simulink model "yek_alef_liang"  (R2024a)
settings: Solver=VariableStepAuto  StartTime=0.0  StopTime=9000  RelTol=1e-3
settings Model: Creator=MAHDI  LastModifiedBy=ASUS
settings SolverCC: AlgebraicLoopSolver=TrustRegion
settings DebuggingCC: UnconnectedInputMsg=warning  UnconnectedOutputMsg=warning  UnconnectedLineMsg=warning
settings ModelReferenceCC: EnableRefExpFcnMdlSchedulingChecks=on
settings RTWCC: GPUComputeCapability=3.5

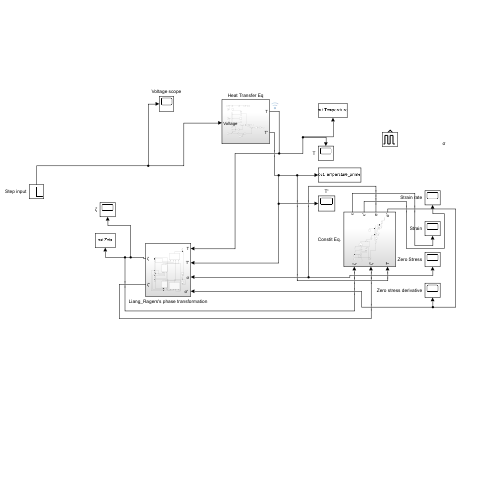
[thumbnail: Simulink's stored preview of the top-level diagram]
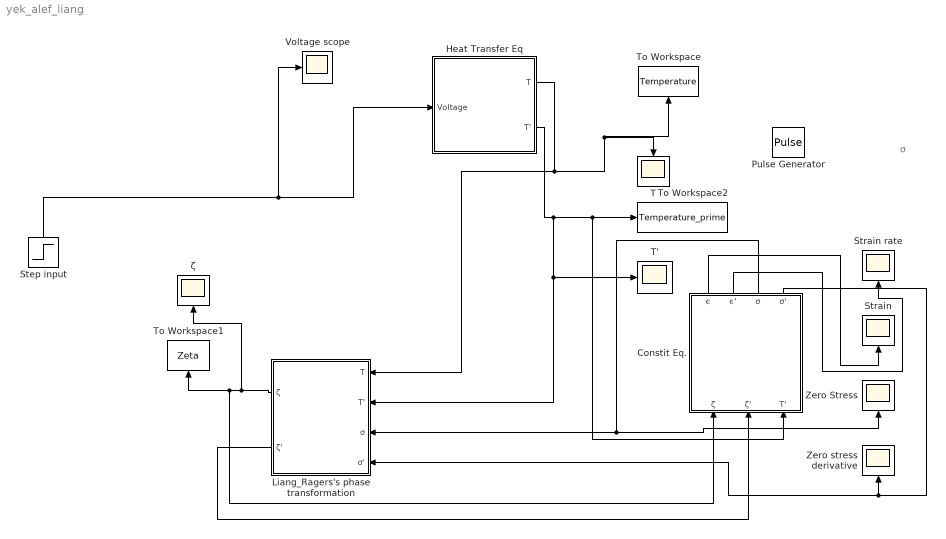
== system yek_alef_liang ==
  note: σ
  Constit Eq. : Subsystem
  Heat Transfer Eq : Subsystem
  Liang_Ragers's phase transformation : Subsystem
  Pulse Generator : DiscretePulseGenerator  PulseType=Time based  Period=100  PulseWidth=5
  Step input : Step  Time=70  Before=1  After=0  SampleTime=0
  Strain : Scope
  Strain rate : Scope
  T : Scope
  T' : Scope
  To Workspace : ToWorkspace  VariableName=Temperature  SampleTime=1
  To Workspace1 : ToWorkspace  VariableName=Zeta  SampleTime=1
  To Workspace2 : ToWorkspace  VariableName=Temperature_prime  SampleTime=1
  Voltage scope : Scope
  Zero Stress : Scope
  Zero stress derivative : Scope
  ζ : Scope
  wires:
  Heat Transfer Eq/1(T) -> To Workspace/1, T/1, Liang_Ragers's phase transformation/1(T)
  Constit Eq./1(ϵ) -> Strain/1
  Step input/1 -> Heat Transfer Eq/1(Voltage), Voltage scope/1
  Heat Transfer Eq/2(T') -> Constit Eq./3(T'), To Workspace2/1, Liang_Ragers's phase transformation/2(T'), T'/1
  Liang_Ragers's phase transformation/1(ζ) -> Constit Eq./1(ζ), To Workspace1/1, ζ/1
  Liang_Ragers's phase transformation/2(ζ') -> Constit Eq./2(ζ')
  Constit Eq./2(ϵ') -> Strain rate/1
  Constit Eq./3(σ) -> Zero Stress/1, Liang_Ragers's phase transformation/3(σ)
  Constit Eq./4(σ') -> Liang_Ragers's phase transformation/4("σ' "), Zero stress derivative/1

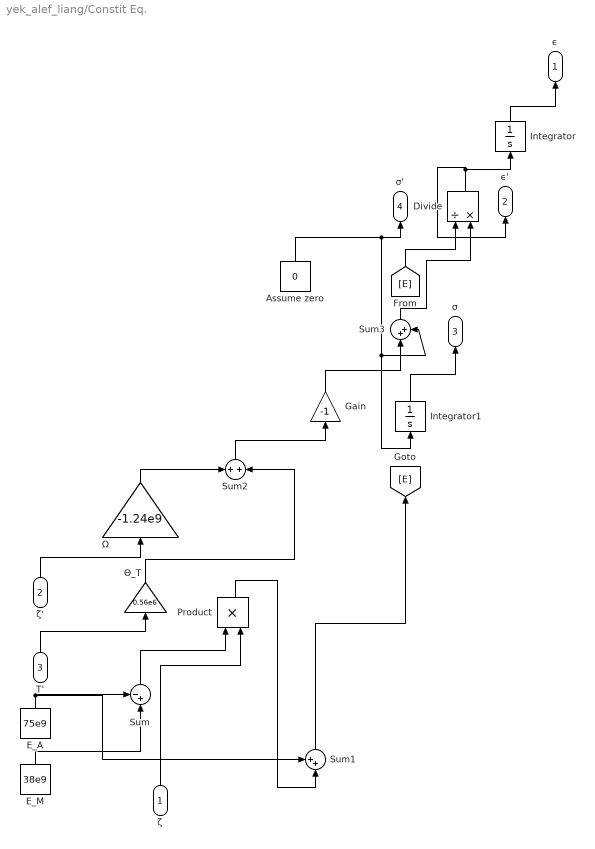
== system yek_alef_liang/Constit Eq. ==
  ζ : Inport
  ζ' : Inport  Port=2
  T' : Inport  Port=3
  Assume zero : Constant  Value=0
  Divide : Product  Inputs=/*
  E_A : Constant  Value=75e9
  E_M : Constant  Value=38e9
  Gain : Gain  Gain=-1
  Integrator : Integrator
  Integrator1 : Integrator
  Product : Product
  Sum : Sum  Inputs=-+|
  Sum1 : Sum  Inputs=++|
  Sum2 : Sum  Inputs=+|+
  Sum3 : Sum  Inputs=|++
  Θ_T : Gain  Gain=0.56e6
  Ω : Gain  Gain=-1.24e9
  ϵ : Outport
  ϵ' : Outport  Port=2
  σ : Outport  Port=3
  σ' : Outport  Port=4
  wires:
  ζ'/1 -> Ω/1
  [E] -> Divide/1
  T'/1 -> Θ_T/1
  Sum3/1 -> Divide/2
  Sum/1 -> Product/1
  E_A/1 -> Sum/1, Sum1/1
  Sum1/1 -> [E]
  Sum2/1 -> Gain/1
  E_M/1 -> Sum/2
  Divide/1 -> ϵ'/1, Integrator/1
  Θ_T/1 -> Sum2/2
  Ω/1 -> Sum2/1
  ζ/1 -> Product/2
  Product/1 -> Sum1/2
  Integrator1/1 -> σ/1
  Assume zero/1 -> Integrator1/1, Sum3/2, σ'/1
  Gain/1 -> Sum3/1
  Integrator/1 -> ϵ/1

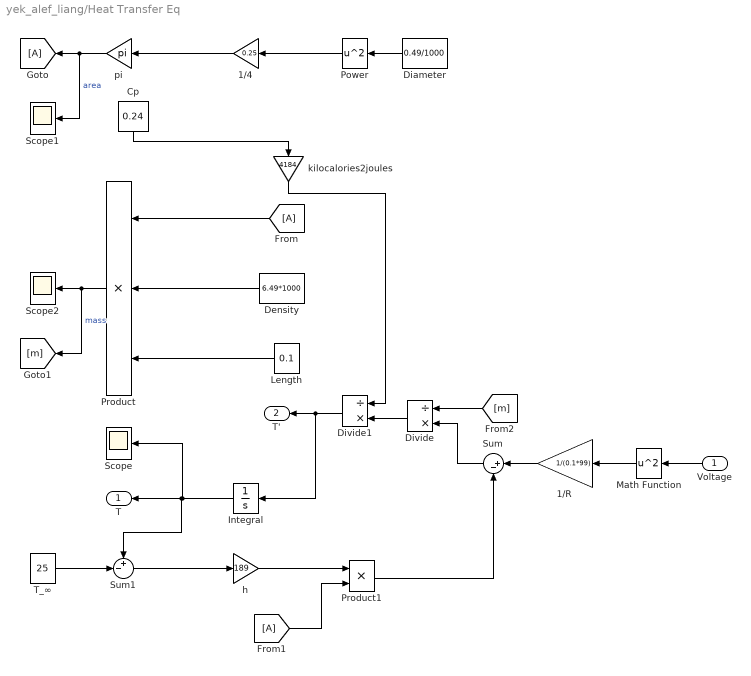
== system yek_alef_liang/Heat Transfer Eq ==
  Voltage : Inport
  1/4 : Gain  Gain=0.25
  1/R : Gain  Gain=1/(0.1*99)
  Cp : Constant  Value=0.24
  Density : Constant  Value=6.49*1000
  Diameter : Constant  Value=0.49/1000
  Divide : Product  Inputs=/*
  Divide1 : Product  Inputs=/*
  From : From
  From1 : From
  Goto : Goto
  Integral : Integrator  InitialCondition=25
  Length : Constant  Value=0.1
  Math Function : Math  Operator=square
  Power : Math  Operator=square
  Product : Product  Inputs=3
  Product1 : Product
  Scope : Scope
  Scope1 : Scope
  Scope2 : Scope
  Sum : Sum  Inputs=|+-
  Sum1 : Sum  Inputs=+-|
  T_∞ : Constant  Value=25
  h : Gain  Gain=189
  "kilocalories2joules " : Gain  Gain=4184
  pi : Gain  Gain=pi
  T : Outport
  T' : Outport  Port=2
  wires:
  Sum/1 -> Divide/2
  Sum1/1 -> h/1
  T_∞/1 -> Sum1/2
  "kilocalories2joules "/1 -> Divide1/1
  Power/1 -> 1/4/1
  Product/1 -> Scope2/1, [m]  "mass"
  pi/1 -> Goto/1, Scope1/1  "area"
  Divide/1 -> Divide1/2
  Diameter/1 -> Power/1
  Divide1/1 -> T'/1, Integral/1
  Cp/1 -> "kilocalories2joules "/1
  1/4/1 -> pi/1
  [m] -> Divide/1
  From/1 -> Product/1
  1/R/1 -> Sum/1
  Density/1 -> Product/2
  Length/1 -> Product/3
  Integral/1 -> Sum1/1, T/1, Scope/1
  Math Function/1 -> 1/R/1
  Product1/1 -> Sum/2
  h/1 -> Product1/1
  From1/1 -> Product1/2
  Voltage/1 -> Math Function/1

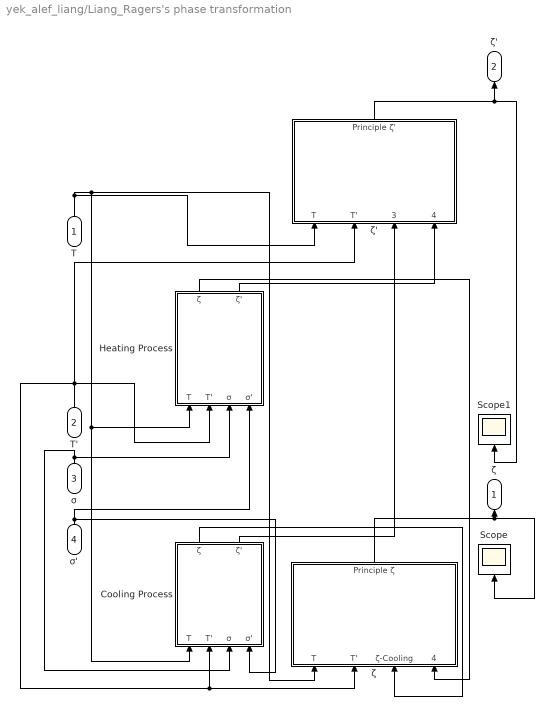
== system yek_alef_liang/Liang_Ragers's phase transformation ==
  T : Inport
  T' : Inport  Port=2
  σ : Inport  Port=3
  "σ' " : Inport  Port=4
  " ζ" : Subsystem
  " ζ'" : Subsystem
  Cooling Process : Subsystem
  Heating Process : Subsystem
  Scope : Scope
  Scope1 : Scope
  ζ : Outport
  ζ' : Outport  Port=2
  wires:
  T'/1 -> " ζ"/2(T'), Cooling Process/2(T'), " ζ'"/2(T'), Heating Process/2(T')
  Heating Process/1(ζ) -> " ζ"/4(ζ- Heating)
  "σ' "/1 -> Cooling Process/4("σ' "), Heating Process/4("σ' ")
  " ζ"/1(Principle ζ) -> ζ/1, Scope/1
  σ/1 -> Cooling Process/3(σ), Heating Process/3(σ)
  T/1 -> Cooling Process/1(T), Heating Process/1(T), " ζ"/1(T), " ζ'"/1(T)
  Heating Process/2(ζ') -> " ζ'"/4(ζ'-Heating)
  Cooling Process/1(ζ) -> " ζ"/3(ζ-Cooling)
  Cooling Process/2(ζ') -> " ζ'"/3(ζ'-Cooling)
  " ζ'"/1(Principle ζ') -> ζ'/1, Scope1/1

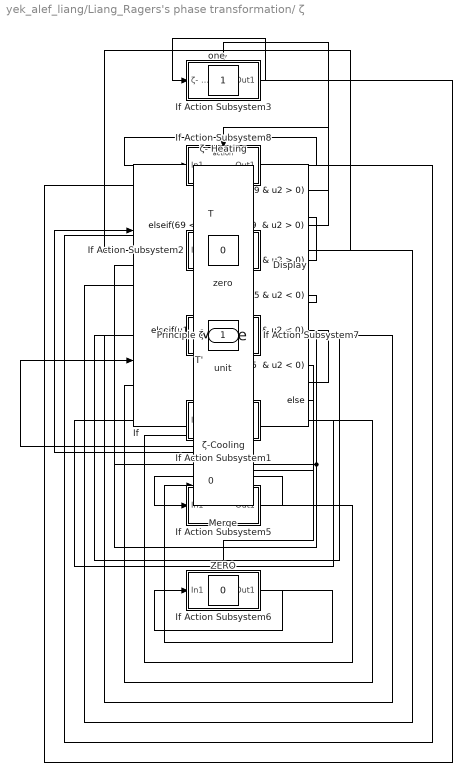
== system yek_alef_liang/Liang_Ragers's phase transformation/ ζ ==
  T : Inport
  T' : Inport  Port=2
  ζ-Cooling : Inport  Port=3
  ζ- Heating : Inport  Port=4
  0 : Constant  Value=0
  Display : Display
  If : If  NumInputs=2  IfExpression=u1 < 69 & u2 > 0  ElseIfExpressions="69 < u1 & u1 < 79  & u2 > 0 , u1 > 79 & u2 > 0 , u1 < 45 & u2 < 0 , u1 > 45 & u1 < 55 & u2 < 0 , u1 > 55  & u2 < 0"
  If Action Subsystem1 : Subsystem  TreatAsAtomicUnit=on
  If Action Subsystem2 : Subsystem  TreatAsAtomicUnit=on
  If Action Subsystem3 : Subsystem  TreatAsAtomicUnit=on
  If Action Subsystem5 : Subsystem  TreatAsAtomicUnit=on
  If Action Subsystem6 : Subsystem  TreatAsAtomicUnit=on
  If Action Subsystem7 : Subsystem  TreatAsAtomicUnit=on
  If Action Subsystem8 : Subsystem  TreatAsAtomicUnit=on
  Merge : Merge  Inputs=7
  ZERO : Constant  Value=0
  one : Constant
  unit : Constant
  zero : Constant  Value=0
  Principle ζ : Outport
  wires:
  T/1 -> If/1
  T'/1 -> If/2
  If/1 -> If Action Subsystem3/Action
  If/2 -> If Action Subsystem8/Action
  If/3 -> If Action Subsystem2/Action
  If/4 -> If Action Subsystem7/Action
  If/5 -> If Action Subsystem1/Action
  If/6 -> If Action Subsystem5/Action
  If/7 -> If Action Subsystem6/Action
  ζ- Heating/1 -> If Action Subsystem8/1(In1)
  0/1 -> If Action Subsystem5/1(In1)
  ZERO/1 -> If Action Subsystem6/1(In1)
  zero/1 -> If Action Subsystem2/1(In1)
  If Action Subsystem7/1(Out1) -> Merge/4
  If Action Subsystem3/1(Out1) -> Merge/1
  If Action Subsystem8/1(Out1) -> Merge/2
  If Action Subsystem2/1(Out1) -> Merge/3
  If Action Subsystem1/1(Out1) -> Merge/5
  If Action Subsystem5/1(Out1) -> Merge/6
  If Action Subsystem6/1(Out1) -> Merge/7
  Merge/1 -> Display/1, Principle ζ/1
  ζ-Cooling/1 -> If Action Subsystem1/1(In1)
  one/1 -> If Action Subsystem3/1(ζ- Heating)
  unit/1 -> If Action Subsystem7/1(ζ-Cooling)

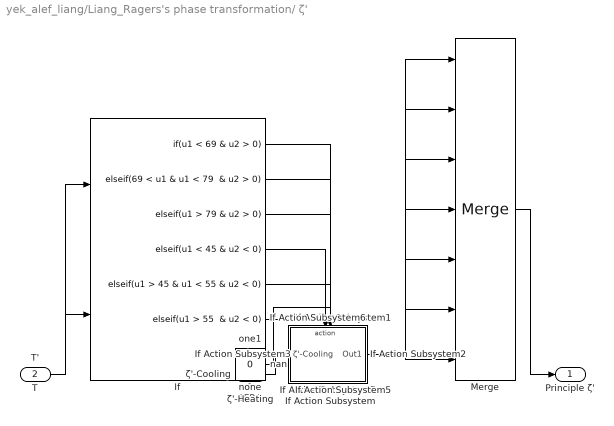
== system yek_alef_liang/Liang_Ragers's phase transformation/ ζ' ==
  T : Inport
  T' : Inport  Port=2
  ζ'-Cooling : Inport  Port=3
  ζ'-Heating : Inport  Port=4
  0 : Constant  Value=0
  If : If  NumInputs=2  IfExpression=u1 < 69 & u2 > 0  ElseIfExpressions="69 < u1 & u1 < 79  & u2 > 0 , u1 > 79 & u2 > 0 , u1 < 45 & u2 < 0 , u1 > 45 & u1 < 55 & u2 < 0 , u1 > 55  & u2 < 0"
  If Action Subsystem : Subsystem  TreatAsAtomicUnit=on
  If Action Subsystem1 : Subsystem  TreatAsAtomicUnit=on
  If Action Subsystem2 : Subsystem  TreatAsAtomicUnit=on
  If Action Subsystem3 : Subsystem  TreatAsAtomicUnit=on
  If Action Subsystem5 : Subsystem  TreatAsAtomicUnit=on
  If Action Subsystem6 : Subsystem  TreatAsAtomicUnit=on
  If Action Subsystem7 : Subsystem  TreatAsAtomicUnit=on
  Merge : Merge  Inputs=7
  ZERO : Constant  Value=0
  nan : Constant  Value=0
  none : Constant  Value=0
  one1 : Constant  Value=0
  Principle ζ' : Outport
  wires:
  ζ'-Heating/1 -> If Action Subsystem1/1(In1)
  If/3 -> If Action Subsystem2/Action
  ζ'-Cooling/1 -> If Action Subsystem3/1(In1)
  If/2 -> If Action Subsystem1/Action
  If/1 -> If Action Subsystem/Action
  T/1 -> If/1
  0/1 -> If Action Subsystem2/1(In1)
  T'/1 -> If/2
  one1/1 -> If Action Subsystem/1(ζ'-Heating)
  If/4 -> If Action Subsystem7/Action
  If/5 -> If Action Subsystem3/Action
  If/6 -> If Action Subsystem5/Action
  If/7 -> If Action Subsystem6/Action
  nan/1 -> If Action Subsystem7/1(ζ'-Cooling)
  none/1 -> If Action Subsystem5/1(In1)
  Merge/1 -> Principle ζ'/1
  ZERO/1 -> If Action Subsystem6/1(In1)
  If Action Subsystem/1(Out1) -> Merge/1
  If Action Subsystem1/1(Out1) -> Merge/2
  If Action Subsystem2/1(Out1) -> Merge/3
  If Action Subsystem7/1(Out1) -> Merge/4
  If Action Subsystem3/1(Out1) -> Merge/5
  If Action Subsystem5/1(Out1) -> Merge/6
  If Action Subsystem6/1(Out1) -> Merge/7

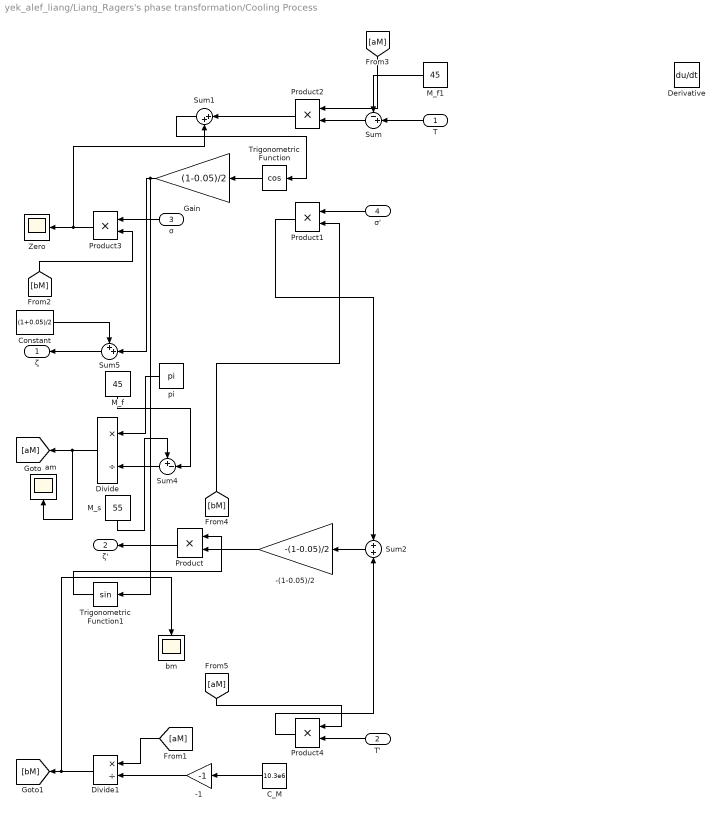
== system yek_alef_liang/Liang_Ragers's phase transformation/Cooling Process ==
  T : Inport
  T' : Inport  Port=2
  σ : Inport  Port=3
  "σ' " : Inport  Port=4
  -(1-0.05)/2 : Gain  Gain=-(1-0.05)/2
  -1 : Gain  Gain=-1
  C_M : Constant  Value=10.3e6
  Constant : Constant  Value=(1+0.05)/2
  Derivative : Derivative
  Divide : Product  Inputs=*/
  Divide1 : Product  Inputs=*/
  Gain : Gain  Gain=(1-0.05)/2
  M_f : Constant  Value=45
  M_f1 : Constant  Value=45
  M_s : Constant  Value=55
  Product{,1..4} (5 alike) : Product
  Sum : Sum  Inputs=-+|
  Sum1 : Sum  Inputs=|++
  Sum2 : Sum  Inputs=+|+
  Sum4 : Sum  Inputs=+-|
  Sum5 : Sum  Inputs=++|
  Trigonometric Function : Trigonometry  Operator=cos
  Trigonometric Function1 : Trigonometry
  Zero : Scope
  am : Scope
  bm : Scope
  pi : Constant  Value=pi
  ζ : Outport
  ζ' : Outport  Port=2
  wires:
  [bM] -> Product3/2
  T/1 -> Sum/2
  Constant/1 -> Sum5/1
  Sum2/1 -> -(1-0.05)/2/1
  Sum/1 -> Product2/2
  Product3/1 -> Zero/1, Sum1/2
  M_s/1 -> Sum4/1
  Product4/1 -> Sum2/2
  Product2/1 -> Sum1/1
  Sum4/1 -> Divide/2
  M_f/1 -> Sum4/2
  Product1/1 -> Sum2/1
  Sum5/1 -> ζ/1
  Divide/1 -> [aM], am/1
  Trigonometric Function1/1 -> Product/1
  Divide1/1 -> [bM], bm/1
  Product/1 -> ζ'/1
  Sum1/1 -> Trigonometric Function/1
  Gain/1 -> Sum5/2, Trigonometric Function1/1
  σ/1 -> Product3/1
  pi/1 -> Divide/1
  [aM] -> Product4/1
  [aM] -> Divide1/1
  -1/1 -> Divide1/2
  [bM] -> Product1/2
  Trigonometric Function/1 -> Gain/1
  -(1-0.05)/2/1 -> Product/2
  C_M/1 -> -1/1
  [aM] -> Product2/1
  "σ' "/1 -> Product1/1
  T'/1 -> Product4/2
  M_f1/1 -> Sum/1

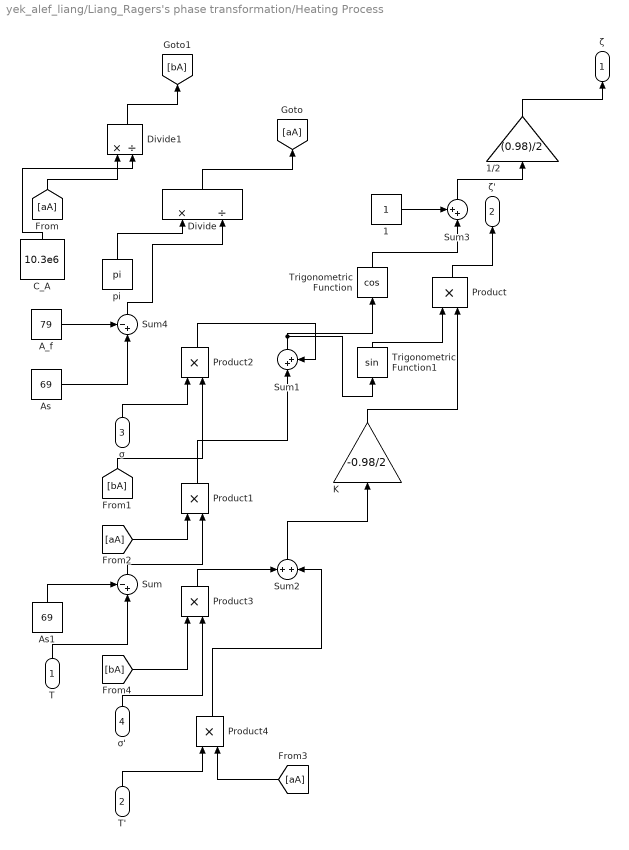
== system yek_alef_liang/Liang_Ragers's phase transformation/Heating Process ==
  T : Inport
  T' : Inport  Port=2
  σ : Inport  Port=3
  "σ' " : Inport  Port=4
  1 : Constant
  1/2 : Gain  Gain=(0.98)/2
  A_f : Constant  Value=79
  As : Constant  Value=69
  As1 : Constant  Value=69
  C_A : Constant  Value=10.3e6
  Divide : Product  Inputs=*/
  Divide1 : Product  Inputs=*/
  K : Gain  Gain=-0.98/2
  Product{,1..4} (5 alike) : Product
  Sum : Sum  Inputs=-+|
  Sum1 : Sum  Inputs=|++
  Sum2 : Sum  Inputs=+|+
  Sum3 : Sum  Inputs=++|
  Sum4 : Sum  Inputs=-+|
  Trigonometric Function : Trigonometry  Operator=cos
  Trigonometric Function1 : Trigonometry
  pi : Constant  Value=pi
  ζ : Outport
  ζ' : Outport  Port=2
  wires:
  Product/1 -> ζ'/1
  Product2/1 -> Sum1/2
  C_A/1 -> Divide1/2
  Divide1/1 -> [bA]
  As1/1 -> Sum/1
  Product1/1 -> Sum1/1
  Divide/1 -> [aA]
  As/1 -> Sum4/2
  A_f/1 -> Sum4/1
  [aA] -> Divide1/1
  T/1 -> Sum/2
  Product4/1 -> Sum2/2
  pi/1 -> Divide/1
  Sum1/1 -> Trigonometric Function/1, Trigonometric Function1/1
  Sum4/1 -> Divide/2
  [aA] -> Product1/1
  σ/1 -> Product2/1
  K/1 -> Product/2
  [bA] -> Product2/2
  Sum2/1 -> K/1
  Product3/1 -> Sum2/1
  Sum/1 -> Product1/2
  1/1 -> Sum3/1
  [bA] -> Product3/1
  [aA] -> Product4/2
  "σ' "/1 -> Product3/2
  T'/1 -> Product4/1
  Trigonometric Function/1 -> Sum3/2
  Trigonometric Function1/1 -> Product/1
  Sum3/1 -> 1/2/1
  1/2/1 -> ζ/1

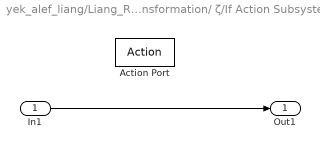
== system yek_alef_liang/Liang_Ragers's phase transformation/ ζ/If Action Subsystem1 ==
  In1 : Inport
  Action Port : ActionPort  ActionPortLabel=elseif( u1 > 45 & u1 < 55 & u2 < 0 )
  Out1 : Outport
  wires:
  In1/1 -> Out1/1

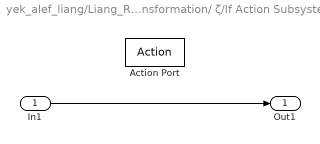
== system yek_alef_liang/Liang_Ragers's phase transformation/ ζ/If Action Subsystem2 ==
  In1 : Inport
  Action Port : ActionPort  ActionPortLabel=elseif( u1 > 79 & u2 > 0 )
  Out1 : Outport
  wires:
  In1/1 -> Out1/1

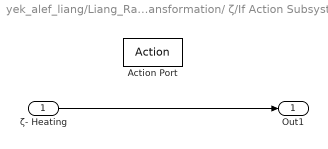
== system yek_alef_liang/Liang_Ragers's phase transformation/ ζ/If Action Subsystem3 ==
  ζ- Heating : Inport
  Action Port : ActionPort  ActionPortLabel=if(u1 < 69 & u2 > 0)
  Out1 : Outport
  wires:
  ζ- Heating/1 -> Out1/1

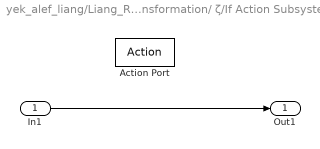
== system yek_alef_liang/Liang_Ragers's phase transformation/ ζ/If Action Subsystem5 ==
  In1 : Inport
  Action Port : ActionPort  ActionPortLabel="elseif( u1 > 55  & u2 < 0)"
  Out1 : Outport
  wires:
  In1/1 -> Out1/1

== system yek_alef_liang/Liang_Ragers's phase transformation/ ζ/If Action Subsystem6 ==
  In1 : Inport
  Action Port : ActionPort  ActionPortLabel=else
  Out1 : Outport
  wires:
  In1/1 -> Out1/1

== system yek_alef_liang/Liang_Ragers's phase transformation/ ζ/If Action Subsystem7 ==
  ζ-Cooling : Inport
  Action Port : ActionPort  ActionPortLabel=elseif( u1 < 45 & u2 < 0 )
  Out1 : Outport
  wires:
  ζ-Cooling/1 -> Out1/1

== system yek_alef_liang/Liang_Ragers's phase transformation/ ζ/If Action Subsystem8 ==
  In1 : Inport
  Action Port : ActionPort  ActionPortLabel="elseif(69 < u1 & u1 < 79  & u2 > 0 )"
  Out1 : Outport
  wires:
  In1/1 -> Out1/1

== system yek_alef_liang/Liang_Ragers's phase transformation/ ζ'/If Action Subsystem ==
  ζ'-Heating : Inport
  Action Port : ActionPort  ActionPortLabel=if(u1 < 69 & u2 > 0)
  Out1 : Outport
  wires:
  ζ'-Heating/1 -> Out1/1

== system yek_alef_liang/Liang_Ragers's phase transformation/ ζ'/If Action Subsystem1 ==
  In1 : Inport
  Action Port : ActionPort  ActionPortLabel="elseif(69 < u1 & u1 < 79  & u2 > 0 )"
  Out1 : Outport
  wires:
  In1/1 -> Out1/1

== system yek_alef_liang/Liang_Ragers's phase transformation/ ζ'/If Action Subsystem2 ==
  In1 : Inport
  Action Port : ActionPort  ActionPortLabel=elseif( u1 > 79 & u2 > 0 )
  Out1 : Outport
  wires:
  In1/1 -> Out1/1

== system yek_alef_liang/Liang_Ragers's phase transformation/ ζ'/If Action Subsystem3 ==
  In1 : Inport
  Action Port : ActionPort  ActionPortLabel=elseif( u1 > 45 & u1 < 55 & u2 < 0 )
  Out1 : Outport
  wires:
  In1/1 -> Out1/1

== system yek_alef_liang/Liang_Ragers's phase transformation/ ζ'/If Action Subsystem5 ==
  In1 : Inport
  Action Port : ActionPort  ActionPortLabel="elseif( u1 > 55  & u2 < 0)"
  Out1 : Outport
  wires:
  In1/1 -> Out1/1

== system yek_alef_liang/Liang_Ragers's phase transformation/ ζ'/If Action Subsystem6 ==
  In1 : Inport
  Action Port : ActionPort  ActionPortLabel=else
  Out1 : Outport
  wires:
  In1/1 -> Out1/1

== system yek_alef_liang/Liang_Ragers's phase transformation/ ζ'/If Action Subsystem7 ==
  ζ'-Cooling : Inport
  Action Port : ActionPort  ActionPortLabel=elseif( u1 < 45 & u2 < 0 )
  Out1 : Outport
  wires:
  ζ'-Cooling/1 -> Out1/1
